simulink model "solar_thermal_parameterized"  (R2024a)
settings: Solver=VariableStepAuto  StartTime=0.0  StopTime=3600*24*3  FixedStep=0.01  RelTol=1e-3
undefined symbols (not defined in the file or in its folder): solar_sig_max, T_design, T_min
libraries: fl_lib x49, nesl_utility x24, SimscapeFluids_lib x1
(part 2 of 2)

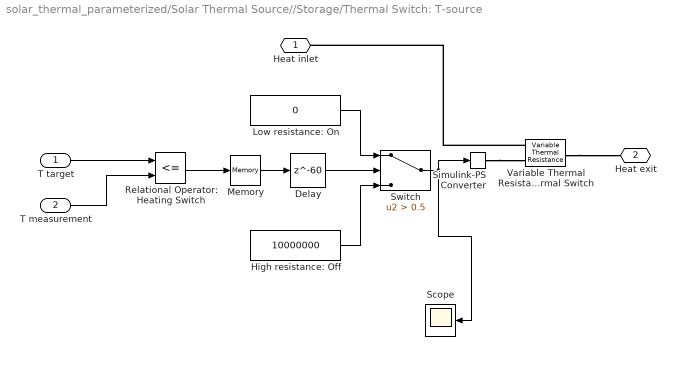
== system solar_thermal_parameterized/Solar Thermal Source//Storage/Thermal Switch: T-source ==
  T target : Inport
  T measurement : Inport  Port=2
  Delay : Delay  DelayLength=60  InitialCondition=0
  High resistance: Off : Constant  Value=10000000
  Low resistance: On : Constant  Value=0
  Memory : Memory
  Relational Operator: Heating Switch : RelationalOperator  Operator=<=  OutDataTypeStr=boolean  RndMeth=Simplest  InputSameDT=off
  Scope : Scope
  Simulink-PS Converter : nesl_utility/Simulink-PS Converter  PhysicalDomain=network_engine_domain  SubClassName=ps_input  LeftPortType=input  RightPortType=output  PseudoPeriodic=off  Frequencies=[]  NoiseDistribution=none  NoiseParameters=[]  Unit=1  AffineConversion=off  FilteringAndDerivatives=provide  SimscapeFilterOrder=1  InputFilterTimeConstant=0.001  UdotUserProvided=0
  Switch : Switch  Criteria=u2 > Threshold  Threshold=0.5  SaturateOnIntegerOverflow=off  InputSameDT=off
  Variable Thermal Resistance: Thermal Switch : fl_lib/Thermal/Thermal Elements/Variable Thermal Resistance  R_min=0 K/W  T_specify=off  T_priority=None  T=0 K  T_nominal_specify=off  T_nominal_value=1  T_nominal_unit=K  Q_specify=off  Q_priority=None  Q=0 W  Q_nominal_specify=off  Q_nominal_value=1  Q_nominal_unit=W
      settings: InternalSimscapePortConfiguration="{\"Bottom\":[],\"Left\":[{\"id\":\"A\",\"label\":\"A\",\"type\":\"foundation.thermal.thermal\"},{\"id\":\"R\",\"label\":\"R\",\"type\":\"input\"}],\"Right\":[{\"id\":\"B\",\"label\":\"B\",\"type\":\"foundation.thermal.thermal\"}],\"Top\":[]}"
  Heat inlet : PMIOPort  Side=Left
  Heat exit : PMIOPort  Port=2  Side=Right
  wires:
  Relational Operator: Heating Switch/1 -> Memory/1
  T measurement/1 -> Relational Operator: Heating Switch/2
  High resistance: Off/1 -> Switch/3
  Switch/1 -> Scope/1, Simulink-PS Converter/1
  T target/1 -> Relational Operator: Heating Switch/1
  Low resistance: On/1 -> Switch/1
  Memory/1 -> Delay/1
  Delay/1 -> Switch/2
  connections:
  Simulink-PS Converter/RConn1 -- Variable Thermal Resistance: Thermal Switch/LConn2
  Variable Thermal Resistance: Thermal Switch/LConn1 -- Heat inlet/RConn1
  Variable Thermal Resistance: Thermal Switch/RConn1 -- Heat exit/RConn1

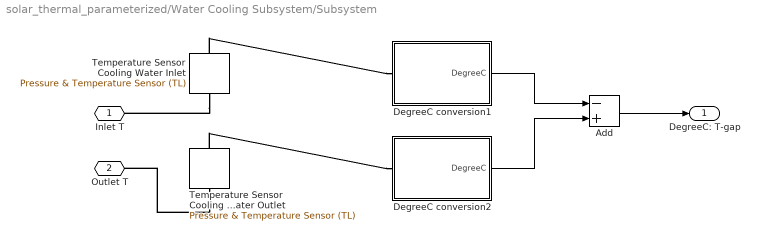
== system solar_thermal_parameterized/Water Cooling Subsystem/Subsystem ==
  Add : Sum  Inputs=-+
  DegreeC conversion1 : Subsystem
  DegreeC conversion2 : Subsystem
  Temperature Sensor Cooling Water Inlet : fl_lib/Thermal Liquid/Sensors/Pressure & Temperature Sensor (TL)  reference=foundation.enum.MeasurementReference.absolute  pressure=false  pressure_spec=foundation.enum.PressureMeasementSpec.Absolute  temperature=true
      settings: InternalSimscapePortConfiguration="{\"Bottom\":[{\"id\":\"T\",\"label\":\"T\",\"type\":\"output\"}],\"Left\":[{\"id\":\"A\",\"label\":\"A\",\"type\":\"foundation.thermal_liquid.thermal_liquid\"}],\"Right\":[],\"Top\":[]}"
  Temperature Sensor Cooling Water Outlet : fl_lib/Thermal Liquid/Sensors/Pressure & Temperature Sensor (TL)  reference=foundation.enum.MeasurementReference.absolute  pressure=false  pressure_spec=foundation.enum.PressureMeasementSpec.Absolute  temperature=true
      settings: InternalSimscapePortConfiguration="{\"Bottom\":[{\"id\":\"T\",\"label\":\"T\",\"type\":\"output\"}],\"Left\":[{\"id\":\"A\",\"label\":\"A\",\"type\":\"foundation.thermal_liquid.thermal_liquid\"}],\"Right\":[],\"Top\":[]}"
  Inlet T : PMIOPort  Side=Left
  Outlet T : PMIOPort  Port=2  Side=Left
  DegreeC: T-gap : Outport
  wires:
  DegreeC conversion1/1(DegreeC) -> Add/1
  DegreeC conversion2/1(DegreeC) -> Add/2
  Add/1 -> DegreeC: T-gap/1
  connections:
  Temperature Sensor Cooling Water Outlet/RConn1 -- DegreeC conversion2/LConn1
  Temperature Sensor Cooling Water Inlet/RConn1 -- DegreeC conversion1/LConn1
  Temperature Sensor Cooling Water Outlet/LConn1 -- Outlet T/RConn1
  Temperature Sensor Cooling Water Inlet/LConn1 -- Inlet T/RConn1

== system solar_thermal_parameterized/Water Cooling Subsystem/Subsystem/DegreeC conversion1 ==
  Absolute zero reference : Constant  Value=-273.15
  PS-Simulink Converter : nesl_utility/PS-Simulink Converter  PhysicalDomain=network_engine_domain  SubClassName=ps_output  LeftPortType=input  RightPortType=output  PseudoPeriodic=off  Frequencies=[]  VectorFormat=inherit  Unit=inherit  AffineConversion=off
  T: degreeC : Sum
  PS-signal : PMIOPort  Side=Left
  DegreeC : Outport
  wires:
  Absolute zero reference/1 -> T: degreeC/2
  PS-Simulink Converter/1 -> T: degreeC/1
  T: degreeC/1 -> DegreeC/1
  connections:
  PS-signal/RConn1 -- PS-Simulink Converter/LConn1

== system solar_thermal_parameterized/Water Cooling Subsystem/Subsystem/DegreeC conversion2 ==
  Absolute zero reference : Constant  Value=-273.15
  PS-Simulink Converter : nesl_utility/PS-Simulink Converter  PhysicalDomain=network_engine_domain  SubClassName=ps_output  LeftPortType=input  RightPortType=output  PseudoPeriodic=off  Frequencies=[]  VectorFormat=inherit  Unit=inherit  AffineConversion=off
  T: degreeC : Sum
  PS-signal : PMIOPort  Side=Left
  DegreeC : Outport
  wires:
  Absolute zero reference/1 -> T: degreeC/2
  PS-Simulink Converter/1 -> T: degreeC/1
  T: degreeC/1 -> DegreeC/1
  connections:
  PS-signal/RConn1 -- PS-Simulink Converter/LConn1
